simulink model "SimpleImpedanceControlConcept"  (R2023b)
settings: Solver=daessc  StartTime=0.0  StopTime=10  RelTol=1e-3
libraries: fl_lib x10, nesl_utility x6, robotcorelib x1, simulink x1
settings Model: Creator=tshifera  LastModifiedBy=fnae
settings OptimizationCC: ReuseModelBlockBuffer=off

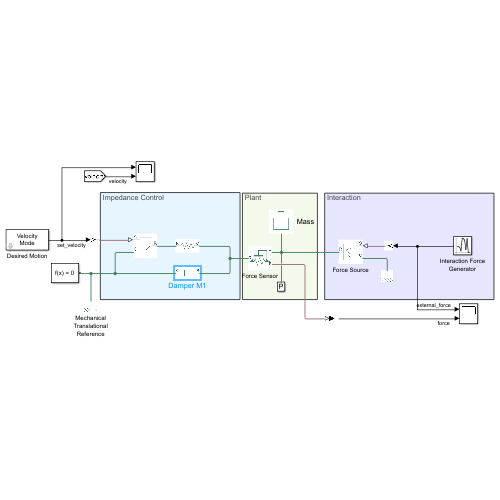
[thumbnail: Simulink's stored preview of the top-level diagram]
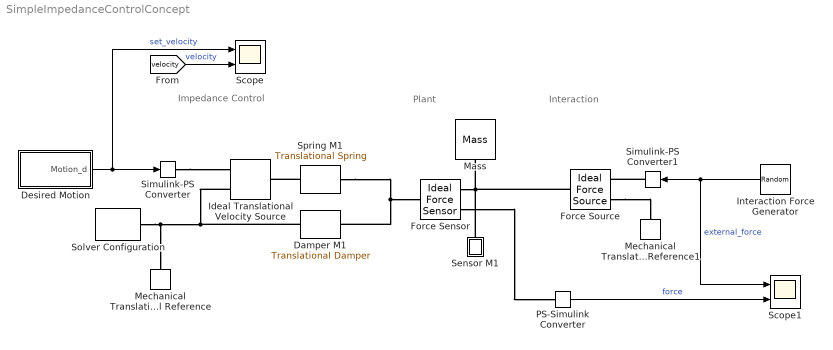
== system SimpleImpedanceControlConcept ==
  note: Plant
  note: Interaction
  note: Impedance Control
  Damper M1 : fl_lib/Mechanical/Translational Elements/Translational Damper  Tag=Factory Generic  D=10 s*N/m  v_specify=off  v_priority=High  v=0 m/s  v_nominal_specify=off  v_nominal_unit=m/s  v_nominal_value=1  f_specify=off  f_priority=High  f=0 N  f_nominal_specify=off  f_nominal_unit=N  f_nominal_value=1
  Desired Motion : Subsystem  mask{desOutput=Velocity, desWP=[ 0, 10, 10, 20, 20, 15], desWPTime=[ 0, 1, 4, 5, 9, 10 ], desWPSpeedLim=zeros( 1, 6 )}
      mask prompts: desOutput "Desired Output"; desWP "Waypoints"; desWPTime "Time"; desWPSpeedLim "Speed Constraint"
      mask TypeOptions desOutput: Position | Velocity
      mask Display:
      | if get_param(gcb,'desOutput') == 'Position'
      |     disp('Position\nMode')
      | else
      |     disp('Velocity\nMode')
      | end
  Force Sensor : fl_lib/Mechanical/Mechanical Sensors/Ideal Force Sensor
  Force Source : fl_lib/Mechanical/Mechanical Sources/Ideal Force Source
  Ideal Translational Velocity Source : fl_lib/Mechanical/Mechanical Sources/Ideal Translational Velocity Source
  Interaction Force Generator : RandomNumber  Variance=20  SampleTime=0.01
  "Mass " : fl_lib/Mechanical/Translational Elements/Mass  Tag=Factory Generic  mass=1 kg  num_ports=foundation.enum.numPorts2.one  v_specify=off  v_priority=High  v=0 m/s  v_nominal_specify=off  v_nominal_unit=m/s  v_nominal_value=1  f_specify=off  f_priority=High  f=0 N  f_nominal_specify=off  f_nominal_unit=N  f_nominal_value=1
  Mechanical Translational Reference : fl_lib/Mechanical/Translational Elements/Mechanical Translational Reference
  Mechanical Translational Reference1 : fl_lib/Mechanical/Translational Elements/Mechanical Translational Reference
  PS-Simulink Converter : nesl_utility/PS-Simulink Converter  PhysicalDomain=network_engine_domain  SubClassName=ps_output  LeftPortType=input  RightPortType=output  PseudoPeriodic=off  Frequencies=[]  VectorFormat=inherit  Unit=inherit  AffineConversion=off
  Scope : Scope  NumInputPorts=2
  Scope1 : Scope  NumInputPorts=2
  Sensor M1 : Subsystem
      mask Display: disp('P')
  Simulink-PS Converter : nesl_utility/Simulink-PS Converter  PhysicalDomain=network_engine_domain  SubClassName=ps_input  LeftPortType=input  RightPortType=output  PseudoPeriodic=off  Frequencies=[]  NoiseDistribution=none  NoiseParameters=[]  Unit=1  AffineConversion=off  FilteringAndDerivatives=provide  SimscapeFilterOrder=1  InputFilterTimeConstant=0.001  UdotUserProvided=0
  Simulink-PS Converter1 : nesl_utility/Simulink-PS Converter  PhysicalDomain=network_engine_domain  SubClassName=ps_input  LeftPortType=input  RightPortType=output  PseudoPeriodic=off  Frequencies=[]  NoiseDistribution=none  NoiseParameters=[]  Unit=1  AffineConversion=off  FilteringAndDerivatives=provide  SimscapeFilterOrder=1  InputFilterTimeConstant=0.001  UdotUserProvided=0
  Solver Configuration : nesl_utility/Solver Configuration  PhysicalDomain=network_engine_domain  SubClassName=solver  LeftPortType=input  RightPortType=generic  Tones=[]  Harmonics=[]  SimulateNoise=off  Profile=off  UseLocalSampling=off  EnableSwitchedLinearOptims=on  FrequencyDomain=off  UseCCode=off  RelTol=0.001  AbsTol=0.001  MinStep=1e-09  ToWorkspace=off  RevertToSquareIcSolve=off  NumHomotopyIterations=100  PhasorMode=off  PhasorModeNumHarmonics=1  ConsistencySolver=NEWTON_XTOL_AFTER_FTOL  IndexReductionMethod=DerivativeReplacement  DoDC=off  ResidualTolerance=1e-09  ConsistencyTolSource=GLOBAL  ConsistencyAbsTol=0.001  ConsistencyRelTol=0.001  ConsistencyTolFactor=0.001  UseLocalSolver=off  LocalSolverChoice=NE_BACKWARD_EULER_ADVANCER  ResolveIndetEquations=on  FunctionEvalNumThread=1  LocalSolverSampleTime=0.001  DoFixedCost=off  MaxNonlinIter=3  MaxModeIter=2  ComputeImpulses=off  ImpulseIterations=2  LinearAlgebra=auto  LinearAlgebraNumThread=0  EquationFormulation=NE_TIME_EF  DelaysMemoryBudget=1024  AutomaticFiltering=on  FilteringTimeConstant=0.001  PartitionStorageMethod=AS_NEEDED  PartitionMemoryBudget=1024  PartitionMethod=ROBUST  MultibodyUseLocalSolver=off  MultibodyLocalSolverChoice=ODE1  MultibodyLocalSolverSampleTime=0.001
  Spring M1 : fl_lib/Mechanical/Translational Elements/Translational Spring  Tag=Factory Generic  spr_rate=200 N/m  v_specify=off  v_priority=High  v=0 m/s  v_nominal_specify=off  v_nominal_unit=m/s  v_nominal_value=1  f_specify=off  f_priority=High  f=0 N  f_nominal_specify=off  f_nominal_unit=N  f_nominal_value=1  x_specify=off  x_priority=High  x=0 m  x_nominal_specify=off  x_nominal_unit=m  x_nominal_value=1
  wires:
  Interaction Force Generator/1 -> Scope1/1, Simulink-PS Converter1/1  "external_force"
  Desired Motion/1(Motion_d) -> Scope/1, Simulink-PS Converter/1  "set_velocity"
  [velocity] -> Scope/2  "velocity"
  PS-Simulink Converter/1 -> Scope1/2  "force"
  connections:
  Solver Configuration/RConn1 -- Mechanical Translational Reference/LConn1 -- Ideal Translational Velocity Source/RConn2 -- Damper M1/RConn1
  Sensor M1/LConn1 -- Force Source/LConn1 -- Force Sensor/RConn1 -- "Mass "/LConn1
  Simulink-PS Converter/RConn1 -- Ideal Translational Velocity Source/RConn1
  Simulink-PS Converter1/RConn1 -- Force Source/RConn1
  Force Source/RConn2 -- Mechanical Translational Reference1/LConn1
  Spring M1/LConn1 -- Ideal Translational Velocity Source/LConn1
  Spring M1/RConn1 -- Force Sensor/LConn1 -- Damper M1/LConn1
  Force Sensor/RConn2 -- PS-Simulink Converter/LConn1

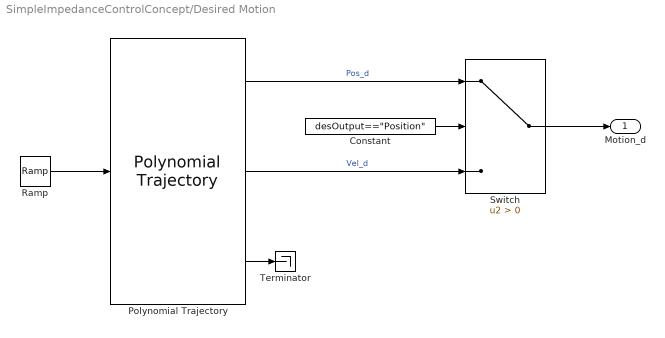
== system SimpleImpedanceControlConcept/Desired Motion ==
  Constant : Constant  Value="desOutput==\"Position\""  OutDataTypeStr=boolean
  Polynomial Trajectory : robotcorelib/Polynomial Trajectory  WaypointSource=Internal  Waypoints=desWP  TimePoints=desWPTime  TimeInterval=[ 1, 4 ]  Method=Cubic Polynomial  ParameterSource=Internal  VelocityBoundaryCondition=desWPSpeedLim  AccelerationBoundaryCondition=zeros( 2, 5 )  SimulateUsing=Interpreted execution
  Ramp : simulink/Sources/Ramp  slope=1  start=0  InitialOutput=0
  Switch : Switch  Criteria=u2 > Threshold  SaturateOnIntegerOverflow=off  InputSameDT=off
  Terminator : Terminator
  Motion_d : Outport
  wires:
  Ramp/1 -> Polynomial Trajectory/1
  Polynomial Trajectory/1 -> Switch/1  "Pos_d"
  Polynomial Trajectory/2 -> Switch/3  "Vel_d"
  Polynomial Trajectory/3 -> Terminator/1
  Constant/1 -> Switch/2
  Switch/1 -> Motion_d/1

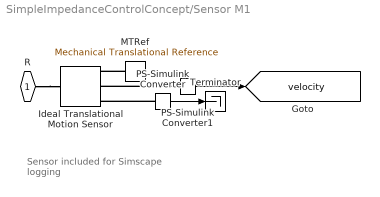
== system SimpleImpedanceControlConcept/Sensor M1 ==
  note: Sensor included for
      | Simscape logging
  Ideal Translational Motion Sensor : fl_lib/Mechanical/Mechanical Sensors/Ideal Translational Motion Sensor  Tag=Factory Generic  reference=foundation.enum.MeasurementReference.difference  acceleration_port=false  velocity_port=true  position_port=true  offset=0 m
  MTRef : fl_lib/Mechanical/Translational Elements/Mechanical Translational Reference  Tag=Factory Generic
  PS-Simulink Converter : nesl_utility/PS-Simulink Converter  PhysicalDomain=network_engine_domain  SubClassName=ps_output  LeftPortType=input  RightPortType=output  PseudoPeriodic=off  Frequencies=[]  VectorFormat=inherit  Unit=inherit  AffineConversion=off
  PS-Simulink Converter1 : nesl_utility/PS-Simulink Converter  PhysicalDomain=network_engine_domain  SubClassName=ps_output  LeftPortType=input  RightPortType=output  PseudoPeriodic=off  Frequencies=[]  VectorFormat=inherit  Unit=inherit  AffineConversion=off
  Terminator : Terminator
  R : PMIOPort  Side=Left
  tag scope: velocity=global
  wires:
  PS-Simulink Converter1/1 -> [velocity]
  PS-Simulink Converter/1 -> Terminator/1
  connections:
  R/RConn1 -- Ideal Translational Motion Sensor/LConn1
  MTRef/LConn1 -- Ideal Translational Motion Sensor/RConn1
  PS-Simulink Converter/LConn1 -- Ideal Translational Motion Sensor/RConn3
  PS-Simulink Converter1/LConn1 -- Ideal Translational Motion Sensor/RConn2
